simulink model "mdaqdemo_fft"  (R2013a)
settings: Solver=FixedStepDiscrete  StartTime=0.0  StopTime=inf  FixedStep=0.0625  RelTol=1e-3
undefined symbols (not defined in the file or in its folder): get
libraries: dspsnks4 x2, dspsrcs4 x1
settings Model: Creator=peselnikmg  LastModifiedBy=skibool
settings OptimizationCC: OptimizeModelRefInitCode=on  LifeSpan=1
settings DebuggingCC: MergeDetectMultiDrivingBlocksExec=error  StrictBusMsg=ErrorOnBusTreatedAsVector  NonBusSignalsTreatedAsBus=error
settings HardwareCC: ProdBitPerLong=40  ProdLargestAtomicInteger=Integer  ProdIntDivRoundTo=Zero  ProdEndianess=LittleEndian  ProdHWDeviceType=Texas Instruments->C6000
settings RTWCC: SystemTargetFile=microdaq.tlc  TemplateMakefile=microdaq.tmf  PostCodeGenCommand=microdaq_postcodegen(buildInfo)  Description=MicroDAQ Real-Time Measurement System  GenerateReport=on  ProcessScript=microdaq_make_rtw_hook  IncludeHyperlinkInReport=on  LaunchReport=on
settings CodeAppCC: IgnoreCustomStorageClasses=off
settings STFCustomTargetCC: CodeReplacementLibrary=TI C674x  CombineOutputUpdateFcns=on  ERTCustomFileBanners=on  SupportContinuousTime=off  SupportNonInlinedSFcns=off  MATLABClassNameForMDSCustomization=Simulink.SoftwareTarget.ERTCustomization  SystemTargetFile=microdaq.tlc
settings ERTTargetCC: CodeReplacementLibrary=TI C674x  GenerateSampleERTMain=off  ParMdlRefBuildCompliant=off  CompOptLevelCompliant=off  ConcurrentExecutionCompliant=off  ERTFirstTimeCompliant=off  ModelStepFunctionPrototypeControlCompliant=off  CPPClassGenCompliant=off  ERTCustomFileTemplate=microdaq_main.tlc

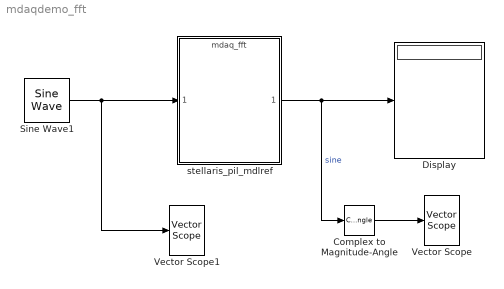
== system mdaqdemo_fft ==
  Complex to Magnitude-Angle : ComplexToMagnitudeAngle  Output=Magnitude
  Display : Display
  Sine Wave1 : dspsrcs4/Sine Wave  Amplitude=1  Frequency=100  Phase=0  SampleMode=Discrete  OutComplex=Real  CompMethod=Trigonometric fcn  TableSize=Speed  SampleTime=1/1024  SamplesPerFrame=64  ResetState=Restart at time zero  dataType=single  wordLen=16  udDataType=sfix(16)  fracBitsMode=Best precision  numFracBits=15  OutDataTypeStr=single  LastOutDataTypeStr=single
  Vector Scope1 : dspsnks4/Vector Scope  ScopeProperties=on  Domain=Time  HorizSpan=1  DisplayProperties=off  AxisGrid=on  Memory=off  FrameNumber=on  AxisLegend=off  AxisZoom=off  OpenScopeAtSimStart=on  OpenScopeImmediately=off  FigPos=get(0,'defaultfigureposition')  AxisProperties=off  XUnits=Hertz  XRange=[0...Fs/2]  InheritXIncr=on  XIncr=1  XLabel=Time  XLimit=Auto  XMin=0  XMax=1  XStart=0  YUnits=dB  YLabel=Amplitude  LineProperties=off  XAxisParamsVer=6.9
      settings: YMin=-10  YMax=10
  Vector Scope : dspsnks4/Vector Scope  ScopeProperties=on  Domain=Frequency  HorizSpan=1  DisplayProperties=off  AxisGrid=on  Memory=off  FrameNumber=on  AxisLegend=off  AxisZoom=off  OpenScopeAtSimStart=on  OpenScopeImmediately=off  FigPos=[68 316 746 527]  AxisProperties=off  XUnits=Hertz  XRange=[0...Fs/2]  InheritXIncr=on  XIncr=1  XLabel=Time  XLimit=User-defined  XMin=0  XMax=512  XStart=0  YUnits=dB  YLabel=Amplitude  LineProperties=off  XAxisParamsVer=6.9
      settings: YMin=-5.6423  YMax=15.665
  stellaris_pil_mdlref : ModelReference  ModelNameDialog=mdaq_fft  SimulationMode=Processor-in-the-loop (PIL)  ModelReferenceVersion=1.27  CopyOfModelName=mdaq_fft  DefaultDataLogging=on
  wires:
  stellaris_pil_mdlref/1 -> Complex to Magnitude-Angle/1, Display/1  "sine"
  Sine Wave1/1 -> Vector Scope1/1, stellaris_pil_mdlref/1
  Complex to Magnitude-Angle/1 -> Vector Scope/1
